simulink model "projets5"  (R2022b)
settings: Solver=FixedStepAuto  StartTime=0.0  StopTime=10.0  RelTol=1e-3  EnableMultiTasking=on
undefined symbols (not defined in the file or in its folder): hw
libraries: raspberrypiAVlib x2
settings Model: Creator=tatan  LastModifiedBy=tatan
settings SolverCC: PositivePriorityOrder=on
settings OptimizationCC: EnhancedBackFolding=on  PassReuseOutputArgsAs=Individual arguments  ZeroExternalMemoryAtStartup=off  ZeroInternalMemoryAtStartup=off  MaxStackSize=64  OptimizeBlockOrder=speed  DifferentSizesBufferReuse=on  OptimizationCustomize=off  EfficientTunableParamExpr=on
settings DebuggingCC: ParameterTunabilityLossMsg=error
settings HardwareCC: ProdBitPerPointer=32  ProdBitPerSizeT=32  ProdBitPerPtrDiffT=32  ProdLargestAtomicInteger=Long  ProdLargestAtomicFloat=Double  ProdWordSize=32  ProdLongLongMode=on  ProdHWDeviceType=ARM Compatible->ARM Cortex  UseEmbeddedCoderFeatures=off  UseSimulinkCoderFeatures=off
settings RTWCC: Description=Embedded Coder  SystemTargetFile=ert.tlc  HardwareBoard=Raspberry Pi  TLCOptions="-aInlineSetEventsForThisBaseRateFcn=TLC_FALSE -aSuppressMultiTaskScheduler=TLC_FALSE  -aRateBasedStepFcn=0"  TemplateMakefile=ert_default_tmf  Toolchain=GNU GCC Embedded Linux  BuildConfiguration=Faster Runs
settings CodeAppCC: ForceParamTrailComments=on  IgnoreCustomStorageClasses=off  OperatorAnnotations=on  SimulinkDataObjDesc=on  SFDataObjDesc=on  InsertBlockDesc=on
settings ERTTargetCC: SupportNonInlinedSFcns=on  SupportVariableSizeSignals=on  ExtModeTransport=2  ExtModeStaticAlloc=on  ExtModeMexFile=ext_xcp  ExtModeIntrfLevel=Level2 - Open

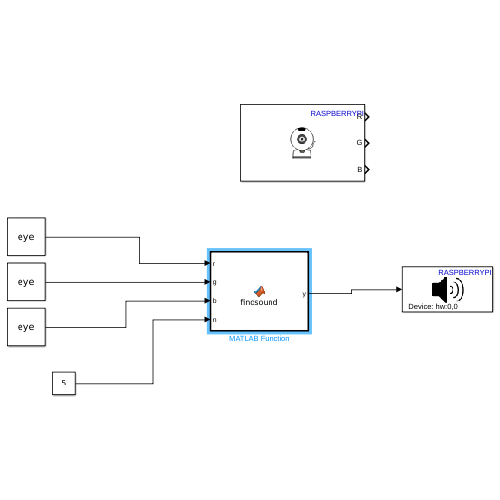
[thumbnail: Simulink's stored preview of the top-level diagram]
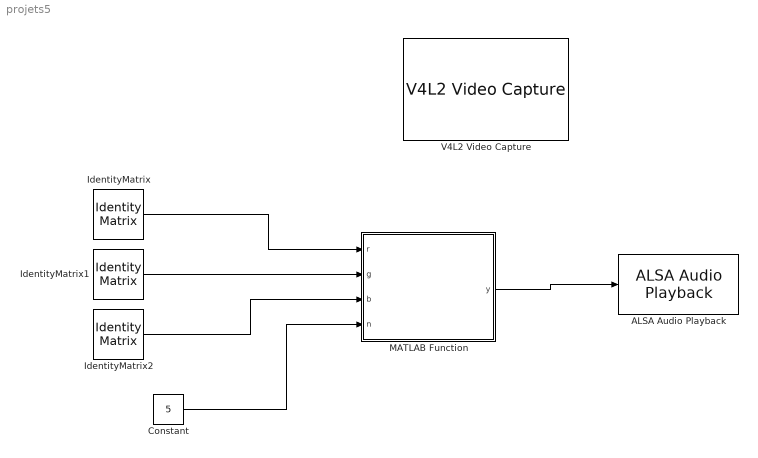
== system projets5 ==
  ALSA Audio Playback : raspberrypiAVlib/ALSA Audio Playback  deviceStr=hw:0,0  sampleRateEnum=44100  queueDuration=0.5  blockPlatform=LINUX
  Constant : Constant  Value=5
  IdentityMatrix : IdentityMatrix  OutputDimensions=160
  IdentityMatrix1 : IdentityMatrix  OutputDimensions=160
  IdentityMatrix2 : IdentityMatrix  OutputDimensions=160
  MATLAB Function : MATLAB Function  TreatAsAtomicUnit=on
  V4L2 Video Capture : raspberrypiAVlib/V4L2 Video Capture  DeviceName=/dev/video0  Resolution=160x120  CustomResolution=[ 320, 240 ]  PixelFormat=RGB  SampleTime=1  pixelOrder=planar  simOutput=Colorbars  imSizeSelection=320x240  imSize=[640, 480]  roi=[0, 0, 640, 480]  m_devName='/dev/video0'  blockPlatform=LINUX  HorizontalFlip=off  VerticalFlip=off  Brightness=0.5  Saturation=0.5  Contrast=0.5  Sharpness=0.5  CameraPan=0  CameraTilt=0  CameraZoom=0.5  EnableManualFocus=on  ManualFocus=0.5
  wires:
  Constant/1 -> MATLAB Function/4(n)
  MATLAB Function/1(y) -> ALSA Audio Playback/1
  IdentityMatrix/1 -> MATLAB Function/1(r)
  IdentityMatrix1/1 -> MATLAB Function/2(g)
  IdentityMatrix2/1 -> MATLAB Function/3(b)

== matlab function projets5/MATLAB Function ==
  settings: sampleTime=1
  data: r input; g input; b input; n input; y output

function y =findsound(r,g,b,n)   
    coder.extrinsic('rgb2ind')
    egf = [0 0];
    egf = size(r);
    s = egf;
    rgb = zeros(s(1,1),s(1,2),3);
    for l=1:s(1,1)
        for c=1:s(1,2)
            rgb(l,c,:) = [r(l,c) g(l,c) b(l,c)];
        end
    end
    %y ok
    %rgb = imresize(rgb,1,"bilinear");
    %rgb = uint16(rgb);
    angle = trouverAngle(rgb, double(n));
    w = pulsation(angle(1));
    t = linspace(0,10,10*int16(2*w));
    bc = t;
    bc = amplitude(angle(1)) * sin(w*t);
    %y=bc;
    y=double(bc(1,8800));
    %y = rgb(1,1);
end


function amp = amplitude(angle)
    amp = abs(angle(1)/90);
end

function w = pulsation(angle)
    w = 440 + (angle / 90) * 220;
end

function angle = trouverAngle(img, n)
    coder.extrinsic('rgb2ind')
    i = findcolor(img,n);
    S = [0 0 0];
    S = size(img);
%     %az = zeros(S(1,1),S(1,2),3);
      [img,map] = rgb2ind(img,n,'nodither');
%     %img = az;
%     imshow(img,map);
     coef = regressionlineair(img, i);
     surete = coef(1,3);%3
     coef = coef(1,2);%2
     coef = 1/coef;
     angle = [-mod(atan(coef)*360/(2*pi),180)+90, surete ];
%     %angle = atan(coef)*360/(2*pi)findcolor
end

function icol = findcolor(img,n)
    coder.extrinsic('rgb2ind')
    %S = [0,0,0];
    %S = size(img);
    %az = zeros(S(1,1),S(1,2),3);
    [img,map] = rgb2ind(img,n,'nodither');
    %az = double(az);
    %img = az;
    index=0;
    minerror = regressionlineair(img,index);
    minerror = minerror(1,3);%3
    for i=1:n-1
        therror = regressionlineair(img,i);
        therror = therror(1,3);%3
        if therror<minerror
            minerror = therror;
            index = i;
        end
    end
    icol = index;
end

function coef = regressionlineair(img, i)
    S = [ 0 0 ];
    coder.extrinsic('regress');
    S = size(img);
    Points = [];
    for l=1:S(1,1)
        int = [0;0];
        int = trouvermilieux(img,l,i);
        Points = [ Points int];
    end
    x = Points(1,:);
    x = transpose(x);
    s = size(x);
    un = ones(s(1,1),1);
    x = [un x];
    x = double(x);
    y = Points(2,:);
    y = transpose(y);
    y = double(y);
    bd = zeros(2,1);
    stats= (double(zeros(1,4)));
    [bd, bint, r, rint, stats] = regress(y,x);
    %autcoef = regress(y,xe)
    %coef = x\y
    be = [transpose(bd) double(stats(1,4))];
    coef = be;
end


function pix = trouvermilieux(img, l, i)
    S = [ 0 0 ];
    S = size(img);
    c = 1;
    temp = [];
    while c<S(1,2)
        px = 0;
        px = double(img(l,c));
        while px~=i & c < S(1,2)
            c=c+1;
            px = double(img(l,c));
        end

        debut = c;
        while px==i & c < S(1,2)
            c=c+1;
            px = double(img(l,c));
        end
        fin = int16(c-1);
        pxd = 0;
        pxd = double(img(l,debut));
        pxf = 0;
        pxf = double(img(l,fin));
        if pxd==i & pxf==i
            vec = [l int16((debut+fin)/2)];
            vec = transpose(vec);
            temp = [ temp vec];
        end
    end
    pix = temp;
end
